simulink model "ltao_v1"  (R2022b)
settings: Solver=FixedStepDiscrete  StartTime=0.0  StopTime=0.6  FixedStep=FEM_Ts  MaxStep=FEM_Ts  RelTol=1e-2
InitFcn:
  | %
  | % Initialization callback function
  | %
  | 
  | try
  |    fprintf('\nGMT IMS version (%s)!\n',simulink_fname );
  | 
  |    % Get Simulink model directory
  |    [filepath,name,ext] = fileparts(which(bdroot));
  | 
  |    if ~strcmp(filepath,pwd)
  |       fprintf('\nChanging current directory to \n %s \n',filepath);
  |       cd(filepath);
  |    end
  | 
  |    %
  |  if(osim.bpless_wl)
  |     fprintf('Generating bumpless wind load time series\n');
  |  end
  | catch
  |    warning('Running the InitFcn from puSimulate script');
  | end
values from neighbouring files (symbols this model uses):
  asm_ssG = XiKL' * asm_ssG * XiKL    [load_ltao_e2e.m]
  Cpi_d = eye(n_Zmodes)* c2d(st.asm.fpi, Ts, c2d_opts)    [evalM2asm_modal.m]    (also in load_ltao_e2e.m = c2d(st.asm.fpi, FEM_Ts, c2d_opts))
  fao_d = c2d(st.glao.fao, st.glao.T, c2d_opts)    [evalM2asm_modal.m]    (also in load_ltao_e2e.m = c2d(st.ltao.fao, FEM_Ts, c2d_opts))
  fao_d4k = c2d(st.ltao.fao, 1/4e3, c2d_opts)    [evalM2asm_modal.m]    (also in load_ltao_e2e.m = c2d(st.ltao.fao, FEM_Ts, c2d_opts))
  FEM_Ts = 1/8e3    (= 0.000125)    [load_ltao_e2e.m]
  fes = c2d(tf((fc_es^2)*4*(pi^2),[1, 2*0.8*fc_es*2*pi, (fc_es^2)*4*(pi^2)]),     st.ltao.T,c2d_opts)    [load_ltao_e2e.m]
  flag_1stOdyn_d = tf(c2d(flag(2,1), Ts, c2d_opts))    [evalM2asm_modal.m]    (also in load_ltao_e2e.m = tf(c2d(flag(2,1),FEM_Ts,c2d_opts)))
  flag_2ndOdyn_d = tf(c2d(flag(3,1), Ts, c2d_opts))    [evalM2asm_modal.m]    (also in load_ltao_e2e.m = tf(c2d(flag(3,1),FEM_Ts,c2d_opts)))
  fpre_d = tf(c2d(st.asm.fpre, Ts, c2d_opts))    [evalM2asm_modal.m]    (also in load_ltao_e2e.m = tf(c2d(fpre,FEM_Ts,c2d_opts)))
  gtt2mnt = eye(2)/(rbm2gtt * Hk_mnt_m1m2)    [load_ltao_e2e.m]
  Hk_mnt_m1m2 = Cm1m2*pinv(Cmnt)    [load_ltao_e2e.m]
  Hpd_d = eye(n_Zmodes)* c2d(st.asm.fpd, Ts, c2d_opts)    [evalM2asm_modal.m]    (also in load_ltao_e2e.m = c2d(st.asm.fpd, FEM_Ts, 'Tustin'))
  Km1rbm_es = (KhpF2es/KhpF2m1rbm)    [load_ltao_e2e.m]
  Ks = cell(7,1)    [load_ltao_e2e.m]
  m1m2_segP_dist = [zeros(42,1); 1e-5*randn(42,1)]    [load_ltao_e2e.m]
  PG = zeros(length(om2),6)    [evalM2asm_modal.m]    (also in load_ltao_e2e.m)
  phiB = inputs2ModalF(mode_ind_vec,indDesInputs) * KinputT    [load_ltao_e2e.m]
  phiC = KoutputT * modalDisp2Outputs(indDesOutputs,mode_ind_vec)    [load_ltao_e2e.m]
  Psi_ss = KoutputT *gainMatrix(indDesOutputs,indDesInputs)* KinputT - K_ss    [load_ltao_e2e.m]
  segPTT2asmCMD = cell(7,1)    [load_ltao_e2e.m]
  Sm1m2_gtt = (Hk_mnt_m1m2*gtt2mnt) * rbm2gtt    [load_ltao_e2e.m]
  st = getcontrol_asm()    [evalM2asm_modal.m]    (also in load_ltao_e2e.m)
undefined symbols (not defined in the file or in its folder): a, az, az_ff_en, b, c, D_seg_piston, D_seg_tt, DiscIntNeverNeededParam, el, fem, gir, m1sys, m2_rbm_dist, m2pos, magnitude, mount, osim, rbm2gtt, Rm1es, Rm2es, sm, VC_modal_stiff
libraries: ims_block_library x7, simulink x2
(part 3 of 3)

== system ltao_v1/Mount_Drv_PDR2021_linear/GIR DT Lugre Fr model/v2z ==
  v : Inport
  g(v) : Inport  Port=2
  z : Inport  Port=3
  Abs : Abs  SaturateOnIntegerOverflow=off
  Divide : Product  Inputs=*/*
  Sum : Sum  Inputs=|+-
  dz : Outport  VectorParamsAs1DForOutWhenUnconnected=off
  wires:
  Abs/1 -> Divide/1
  Divide/1 -> Sum/2
  v/1 -> Sum/1, Abs/1
  Sum/1 -> dz/1
  g(v)/1 -> Divide/2
  z/1 -> Divide/3

== system ltao_v1/Mount_Drv_PDR2021_linear/Parasitic torques model /AZ_Parasitic_Torque ==
  Drive_Pos : Inport
  Drive_Torque : Inport  Port=2
  Cogging : Lookup_n-D  NumberOfTableDimensions=1  LookupTableObject=F_ripple  BreakpointsForDimension1=ParasiticModelStruc.Pos  Table=ParasiticModelStruc.oCog.Amp  InternalRulePriority=Speed  RndMeth=Simplest
  Constant : Constant  Value=0.1869
  Divide : Product  Inputs=**
  EMF Distortion : Lookup_n-D  NumberOfTableDimensions=1  LookupTableObject=F_ripple  BreakpointsForDimension1=ParasiticModelStruc.Pos  Table=ParasiticModelStruc.oEmf.Amp  InternalRulePriority=Speed  RndMeth=Simplest
  Gain : Gain  Gain=1/ParasiticModelStruc.R
  Gain1 : Gain  Gain=1/250
  Gain2 : Gain  Gain=1/ParasiticModelStruc.N_Segm
  Mod : Math  Operator=rem  SignedPower=on
  Mod1 : Math  Operator=rem  SignedPower=on
  Radius : Gain  Gain=ParasiticModelStruc.R
  Sum1 : Sum
  Sum2 : Sum
  Parasitic_Torque : Outport  VectorParamsAs1DForOutWhenUnconnected=off
  wires:
  Divide/1 -> Sum1/1
  Gain1/1 -> Gain2/1  "I_rms"
  Mod1/1 -> EMF Distortion/1, Cogging/1
  Cogging/1 -> Sum1/2
  Radius/1 -> Mod/1  "driven  distance"
  Drive_Torque/1 -> Gain/1
  Gain/1 -> Gain1/1  "Force"
  EMF Distortion/1 -> Divide/2
  Sum2/1 -> Mod1/1
  Mod/1 -> Sum2/1
  Gain2/1 -> Divide/1  "I_rms pro Segment"
  Constant/1 -> Mod/2, Sum2/2, Mod1/2
  Drive_Pos/1 -> Radius/1  "Drive Position"
  Sum1/1 -> Parasitic_Torque/1

== system ltao_v1/Mount_Drv_PDR2021_linear/Parasitic torques model /EL_Parasitic_Torque ==
  Drive_Pos : Inport
  Drive_Torque : Inport  Port=2
  Cogging : Lookup_n-D  NumberOfTableDimensions=1  LookupTableObject=F_ripple  BreakpointsForDimension1=ParasiticModelStruc.Pos  Table=ParasiticModelStruc.oCog.Amp  InternalRulePriority=Speed  RndMeth=Simplest
  Constant : Constant  Value=0.1869
  Divide : Product  Inputs=**
  EMF Distortion : Lookup_n-D  NumberOfTableDimensions=1  LookupTableObject=F_ripple  BreakpointsForDimension1=ParasiticModelStruc.Pos  Table=ParasiticModelStruc.oEmf.Amp  InternalRulePriority=Speed  RndMeth=Simplest
  Gain : Gain  Gain=1/ParasiticModelStruc.R
  Gain1 : Gain  Gain=1/250
  Gain2 : Gain  Gain=1/ParasiticModelStruc.N_Segm
  Mod : Math  Operator=rem  SignedPower=on
  Mod1 : Math  Operator=rem  SignedPower=on
  Radius : Gain  Gain=ParasiticModelStruc.R
  Sum1 : Sum
  Sum2 : Sum
  Parasitic_Torque : Outport  VectorParamsAs1DForOutWhenUnconnected=off
  wires:
  Sum1/1 -> Parasitic_Torque/1
  Drive_Torque/1 -> Gain/1
  EMF Distortion/1 -> Divide/2
  Drive_Pos/1 -> Radius/1  "Drive Position"
  Gain1/1 -> Gain2/1  "I_rms"
  Gain2/1 -> Divide/1  "I_rms pro Segment"
  Gain/1 -> Gain1/1  "Force"
  Mod/1 -> Sum2/1
  Cogging/1 -> Sum1/2
  Radius/1 -> Mod/1  "driven  distance"
  Sum2/1 -> Mod1/1
  Mod1/1 -> EMF Distortion/1, Cogging/1
  Divide/1 -> Sum1/1
  Constant/1 -> Mod/2, Sum2/2, Mod1/2

== system ltao_v1/Mount_Drv_PDR2021_linear/Parasitic torques model /GIR_Parasitic_Torque ==
  note: EMF Torque Model
  note: Cogging Torque Model
  Drive_Pos : Inport
  Drive_Torque : Inport  Port=2
  CogAmp : Constant  Value=ParasiticModelStruc.oCog.amp
  CogSpatFreq : Constant  Value=ParasiticModelStruc.oCog.sfr
  Product : Product
  Product1 : Product  RndMeth=Zero
  Product2 : Product  Inputs=3  RndMeth=Zero
  Product3 : Product  RndMeth=Zero
  Product4 : Product  RndMeth=Zero
  RippleAmpFactor : Constant  Value=ParasiticModelStruc.oEmf.ampFact
  RippleSpatFreq : Constant  Value=ParasiticModelStruc.oEmf.sfr
  Sign : Signum
  Sum : Sum  Inputs=|++
  Sum1 : Sum  Inputs=++|
  ToPretension : Constant  Value=T_pretension
  Trigonometric Function : Trigonometry
  Trigonometric Function1 : Trigonometry
  Parasitic_Torque : Outport  VectorParamsAs1DForOutWhenUnconnected=off
  wires:
  RippleAmpFactor/1 -> Product2/2
  Product1/1 -> Trigonometric Function/1
  RippleSpatFreq/1 -> Product1/2
  Product3/1 -> Trigonometric Function1/1
  Trigonometric Function1/1 -> Product4/1
  CogSpatFreq/1 -> Product3/2
  Drive_Pos/1 -> Product3/1, Product1/1  "Drive Position"
  CogAmp/1 -> Product4/2
  Product4/1 -> Sum/2
  Product2/1 -> Sum/1
  Sum/1 -> Parasitic_Torque/1
  Trigonometric Function/1 -> Product2/3
  Sum1/1 -> Product2/1
  Drive_Torque/1 -> Sign/1, Sum1/2  "Drive Torque (Nm)"
  Sign/1 -> Product/2
  ToPretension/1 -> Product/1
  Product/1 -> Sum1/1

== system ltao_v1/Mount_Drv_PDR2021_linear/Parasitic torques model /Subsystem ==
  Az Pos : Inport
  Az To : Inport  Port=2
  El Pos : Inport  Port=3
  El To : Inport  Port=4
  Gir Pos : Inport  Port=5
  Gir To : Inport  Port=6
  Constant2 : Constant
  Demux1 : Demux  Outputs=3
  Mux1 : Mux  Inputs=3
  Mux7 : Mux  Inputs=3
  Parasitic Torques : Subsystem
  Out1 : Outport  VectorParamsAs1DForOutWhenUnconnected=off
  Out2 : Outport  Port=2  VectorParamsAs1DForOutWhenUnconnected=off
  Out3 : Outport  Port=3  VectorParamsAs1DForOutWhenUnconnected=off
  wires:
  Demux1/1 -> Out1/1
  Demux1/2 -> Out2/1
  Gir Pos/1 -> Mux7/3
  Demux1/3 -> Out3/1
  Az Pos/1 -> Mux7/1
  Mux7/1 -> Parasitic Torques/2(MotPos)
  Mux1/1 -> Parasitic Torques/1(MotTo)
  Constant2/1 -> Parasitic Torques/Enable
  El Pos/1 -> Mux7/2
  Parasitic Torques/1(ParasiticTo) -> Demux1/1
  Az To/1 -> Mux1/1
  El To/1 -> Mux1/2
  Gir To/1 -> Mux1/3

== system ltao_v1/Telescope model/Structural Dynamics GMT/FEM_SS ==
  note: 2nd order form simulation
  In : Inport
  Mount vel gnd : Terminator  Commented=on
  Sum2 : Sum  Inputs=+++
  Sum3 : Sum  Inputs=+++
  Unit Delay : UnitDelay  SampleTime=FEM_Ts  HasFrameUpgradeWarning=on
  Unit Delay1 : UnitDelay  SampleTime=FEM_Ts  HasFrameUpgradeWarning=on
  gamma1 : Gain  Gain=PG(:,3)
  gamma2 : Gain  Gain=PG(:,6)
  phi11 : Gain  Gain=PG(:,1)
  phi12 : Gain  Gain=PG(:,2)
  phi21 : Gain  Gain=PG(:,4)
  phi22 : Gain  Gain=PG(:,5)
  phiB : Gain  Gain=phiB  Multiplication=Matrix(K*u) (u vector)
  phiC : Gain  Gain=phiC  Multiplication=Matrix(K*u) (u vector)
  phiCv : Gain  Gain=phiC(1:14,:)  Multiplication=Matrix(K*u) (u vector)
  pos : Outport  VectorParamsAs1DForOutWhenUnconnected=off
  mount_vel : Outport  Port=2  VectorParamsAs1DForOutWhenUnconnected=off
  wires:
  phiCv/1 -> Mount vel gnd/1, mount_vel/1
  In/1 -> phiB/1
  phiC/1 -> pos/1
  phiB/1 -> gamma1/1, gamma2/1
  Unit Delay1/1 -> phi22/1, phi12/1, phiCv/1
  phi11/1 -> Sum3/3
  gamma1/1 -> Sum3/1
  phi22/1 -> Sum2/1
  phi21/1 -> Sum2/2
  gamma2/1 -> Sum2/3
  Sum3/1 -> Unit Delay/1
  Sum2/1 -> Unit Delay1/1
  phi12/1 -> Sum3/2
  Unit Delay/1 -> phiC/1, phi21/1, phi11/1

== system ltao_v1/Telescope model/Structural Dynamics GMT_/FEM_SS ==
  note: 2nd order form simulation
  In : Inport
  Mount vel gnd : Terminator  Commented=on
  Sum2 : Sum  Inputs=+++
  Sum3 : Sum  Inputs=+++
  Unit Delay : UnitDelay  SampleTime=FEM_Ts  HasFrameUpgradeWarning=on
  Unit Delay1 : UnitDelay  SampleTime=FEM_Ts  HasFrameUpgradeWarning=on
  gamma1 : Gain  Gain=PG(:,3)
  gamma2 : Gain  Gain=PG(:,6)
  phi11 : Gain  Gain=PG(:,1)
  phi12 : Gain  Gain=PG(:,2)
  phi21 : Gain  Gain=PG(:,4)
  phi22 : Gain  Gain=PG(:,5)
  phiB : Gain  Gain=phiB  Multiplication=Matrix(K*u) (u vector)
  phiC : Gain  Gain=phiC  Multiplication=Matrix(K*u) (u vector)
  phiCv : Gain  Gain=phiC(1:14,:)  Multiplication=Matrix(K*u) (u vector)
  pos : Outport  VectorParamsAs1DForOutWhenUnconnected=off
  mount_vel : Outport  Port=2  VectorParamsAs1DForOutWhenUnconnected=off
  wires:
  Unit Delay/1 -> phi11/1, phi21/1, phiC/1
  phi12/1 -> Sum3/2
  Sum2/1 -> Unit Delay1/1
  Sum3/1 -> Unit Delay/1
  gamma2/1 -> Sum2/3
  phi21/1 -> Sum2/2
  phi22/1 -> Sum2/1
  gamma1/1 -> Sum3/1
  phi11/1 -> Sum3/3
  Unit Delay1/1 -> phiCv/1, phi12/1, phi22/1
  phiB/1 -> gamma2/1, gamma1/1
  phiC/1 -> pos/1
  In/1 -> phiB/1
  phiCv/1 -> mount_vel/1, Mount vel gnd/1

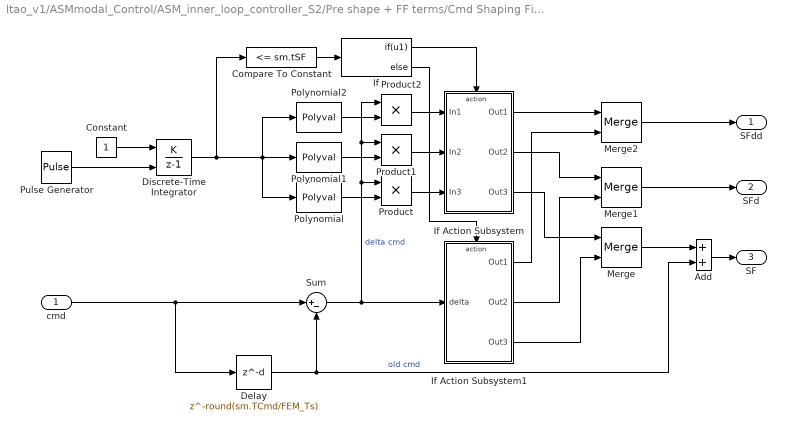
== system ltao_v1/ASMmodal_Control/ASM_inner_loop_controller_S2/Pre shape + FF terms/Cmd Shaping Filter ==
  cmd : Inport
  Add : Sum
  Compare To Constant : simulink/Logic and Bit Operations/Compare To Constant  relop=<=  const=sm.tSF  OutDataTypeStr=boolean
  Constant : Constant
  Delay : Delay  DelayLength=round(sm.TCmd/FEM_Ts)
  Discrete-Time Integrator : DiscreteIntegrator  IntegratorMethod=Accumulation: Forward Euler  gainval=FEM_Ts  ExternalReset=rising  SampleTime=FEM_Ts  ICPrevOutput=DiscIntNeverNeededParam  ICPrevScaledInput=DiscIntNeverNeededParam
  If : If  IfExpression=u1
  If Action Subsystem : Subsystem  TreatAsAtomicUnit=on
  If Action Subsystem1 : Subsystem  TreatAsAtomicUnit=on
  Merge : Merge
  Merge1 : Merge
  Merge2 : Merge
  Polynomial : Polyval  Coefs=[sm.d3SF/20, sm.d2SF/12, sm.d1SF/6, 0, 0, 0]
  Polynomial1 : Polyval  Coefs=[5*sm.d3SF/20, 4*sm.d2SF/12, 3*sm.d1SF/6, 0, 0]
  Polynomial2 : Polyval  Coefs=[20*sm.d3SF/20, 12*sm.d2SF/12, 6*sm.d1SF/6, 0]
  Product : Product
  Product1 : Product
  Product2 : Product
  Pulse Generator : DiscretePulseGenerator  Period=round(sm.TCmd/FEM_Ts)  SampleTime=FEM_Ts
  Sum : Sum  Inputs=|+-
  SFdd : Outport  VectorParamsAs1DForOutWhenUnconnected=off
  SFd : Outport  Port=2  VectorParamsAs1DForOutWhenUnconnected=off
  SF : Outport  Port=3  VectorParamsAs1DForOutWhenUnconnected=off
  wires:
  Discrete-Time Integrator/1 -> Compare To Constant/1, Polynomial2/1, Polynomial/1, Polynomial1/1
  Constant/1 -> Discrete-Time Integrator/1
  Polynomial1/1 -> Product1/2
  Polynomial/1 -> Product/2
  Polynomial2/1 -> Product2/2
  Sum/1 -> If Action Subsystem1/1(delta), Product2/1, Product1/1, Product/1  "delta cmd"
  Add/1 -> SF/1
  Compare To Constant/1 -> If/1
  Product/1 -> If Action Subsystem/3(In3)
  Product1/1 -> If Action Subsystem/2(In2)
  Product2/1 -> If Action Subsystem/1(In1)
  Merge1/1 -> SFd/1
  Merge/1 -> Add/1
  Delay/1 -> Sum/2, Add/2  "old cmd"
  If/1 -> If Action Subsystem/Action
  If/2 -> If Action Subsystem1/Action
  Merge2/1 -> SFdd/1
  If Action Subsystem/1(Out1) -> Merge2/1
  If Action Subsystem1/1(Out1) -> Merge2/2
  If Action Subsystem/2(Out2) -> Merge1/1
  If Action Subsystem/3(Out3) -> Merge/1
  If Action Subsystem1/2(Out2) -> Merge1/2
  If Action Subsystem1/3(Out3) -> Merge/2
  Pulse Generator/1 -> Discrete-Time Integrator/2
  cmd/1 -> Delay/1, Sum/1

== system ltao_v1/Mount_Drv_PDR2021_linear/AZ DT Lugre Fr model/g(v)/gs ==
  v : Inport
  Enable : EnablePort
  Divide : Product  Inputs=**
  Gain : Gain  Gain=1/frParStruct.vs
  Math Function : Math  SignedPower=on
  Math Function1 : Math  Operator=magnitude^2  SignedPower=on
  Sum : Sum  Inputs=|++
  Unary Minus : UnaryMinus
  gc : Constant  Value=frParStruct.Tc/frParStruct.sigm0
  gs : Constant  Value=(frParStruct.Ts-frParStruct.Tc)/frParStruct.sigm0
  gs(v) : Outport  VectorParamsAs1DForOutWhenUnconnected=off
  wires:
  Math Function/1 -> Divide/1
  gs/1 -> Divide/2
  Math Function1/1 -> Unary Minus/1
  Unary Minus/1 -> Math Function/1
  Gain/1 -> Math Function1/1
  v/1 -> Gain/1
  gc/1 -> Sum/2
  Divide/1 -> Sum/1
  Sum/1 -> gs(v)/1

== system ltao_v1/Mount_Drv_PDR2021_linear/EL DT Lugre Fr model/g(v)/gs ==
  v : Inport
  Enable : EnablePort
  Divide : Product  Inputs=**
  Gain : Gain  Gain=1/frParStruct.vs
  Math Function : Math  SignedPower=on
  Math Function1 : Math  Operator=magnitude^2  SignedPower=on
  Unary Minus : UnaryMinus
  gs : Constant  Value=(frParStruct.Ts-frParStruct.Tc)/frParStruct.sigm0
  gs(v) : Outport  VectorParamsAs1DForOutWhenUnconnected=off
  wires:
  Math Function/1 -> Divide/1
  gs/1 -> Divide/2
  Math Function1/1 -> Unary Minus/1
  Unary Minus/1 -> Math Function/1
  Gain/1 -> Math Function1/1
  v/1 -> Gain/1
  Divide/1 -> gs(v)/1

== system ltao_v1/Mount_Drv_PDR2021_linear/GIR DT Lugre Fr model/g(v)/gs ==
  v : Inport
  Enable : EnablePort
  Divide : Product  Inputs=**
  Gain : Gain  Gain=1/frParStruct.vs
  Math Function : Math  SignedPower=on
  Math Function1 : Math  Operator=magnitude^2  SignedPower=on
  Unary Minus : UnaryMinus
  gs : Constant  Value=(frParStruct.Ts-frParStruct.Tc)/frParStruct.sigm0
  gs(v) : Outport  VectorParamsAs1DForOutWhenUnconnected=off
  wires:
  Math Function/1 -> Divide/1
  gs/1 -> Divide/2
  Math Function1/1 -> Unary Minus/1
  Unary Minus/1 -> Math Function/1
  Gain/1 -> Math Function1/1
  v/1 -> Gain/1
  Divide/1 -> gs(v)/1

== system ltao_v1/Mount_Drv_PDR2021_linear/Parasitic torques model /Subsystem/Parasitic Torques ==
  MotTo : Inport
  MotPos : Inport  Port=2
  Enable : EnablePort
  Demux1 : Demux  Outputs=2
  Demux2 : Demux  Outputs=2
  Demux3 : Demux  Outputs=2
  Mux2 : Mux  Inputs=2
  Mux3 : Mux  Inputs=3
  Parasitic AZ : Subsystem  mask{Pos=az.oParasitic.Pos, Amp_Cog=az.oParasitic.oCog.Amp, Amp_EMF=az.oParasitic.oEmf.Amp, R=az.oParasitic.R, N_Segm=az.oParasitic.N_Segm}
  Parasitic EL : Subsystem  mask{Pos=el.oParasitic.Pos, Amp_Cog=el.oParasitic.oCog.Amp, Amp_EMF=el.oParasitic.oEmf.Amp, R=el.oParasitic.R, N_Segm=el.oParasitic.N_Segm}
  Parasitic GIR : Subsystem  mask{cog_sfr=gir.oParasitic.oCog.sfr, cog_amp=gir.oParasitic.oCog.amp, emf_sfr=gir.oParasitic.oEmf.sfr, emf_ampFact=gir.oParasitic.oEmf.ampFact, T_pretension=gir.T_pretension}
  Sel : Selector  InputPortWidth=6  IndexOptions=Index vector (dialog)  Indices=[1 4]  OutputSizes=1
  Sel1 : Selector  InputPortWidth=6  IndexOptions=Index vector (dialog)  Indices=[2 5]  OutputSizes=1
  Sel2 : Selector  InputPortWidth=6  IndexOptions=Index vector (dialog)  Indices=[3 6]  OutputSizes=1
  ParasiticTo : Outport
  wires:
  Mux3/1 -> ParasiticTo/1
  Mux2/1 -> Sel/1, Sel2/1, Sel1/1
  MotTo/1 -> Mux2/1
  MotPos/1 -> Mux2/2
  Sel/1 -> Demux3/1
  Demux3/2 -> Parasitic AZ/2(MotPos)
  Parasitic AZ/1(To) -> Mux3/1
  Sel1/1 -> Demux1/1
  Demux1/2 -> Parasitic EL/2(MotPos)
  Parasitic EL/1(To) -> Mux3/2
  Demux2/1 -> Parasitic GIR/1(MotTo)
  Demux2/2 -> Parasitic GIR/2(MotPos)
  Sel2/1 -> Demux2/1
  Demux3/1 -> Parasitic AZ/1(MotTo)
  Demux1/1 -> Parasitic EL/1(MotTo)
  Parasitic GIR/1(To) -> Mux3/3

== system ltao_v1/ASMmodal_Control/ASM_inner_loop_controller_S2/Pre shape + FF terms/Cmd Shaping Filter/If Action Subsystem ==
  In1 : Inport
  In2 : Inport  Port=2
  In3 : Inport  Port=3
  Action Port : ActionPort
  Out1 : Outport  VectorParamsAs1DForOutWhenUnconnected=off
  Out2 : Outport  Port=2  VectorParamsAs1DForOutWhenUnconnected=off
  Out3 : Outport  Port=3  VectorParamsAs1DForOutWhenUnconnected=off
  wires:
  In1/1 -> Out1/1
  In2/1 -> Out2/1
  In3/1 -> Out3/1

== system ltao_v1/ASMmodal_Control/ASM_inner_loop_controller_S2/Pre shape + FF terms/Cmd Shaping Filter/If Action Subsystem1 ==
  delta : Inport
  Action Port : ActionPort
  Gain : Gain  Gain=0
  Out1 : Outport  VectorParamsAs1DForOutWhenUnconnected=off
  Out2 : Outport  Port=2  VectorParamsAs1DForOutWhenUnconnected=off
  Out3 : Outport  Port=3  VectorParamsAs1DForOutWhenUnconnected=off
  wires:
  delta/1 -> Gain/1, Out3/1
  Gain/1 -> Out1/1, Out2/1

== system ltao_v1/Mount_Drv_PDR2021_linear/Parasitic torques model /Subsystem/Parasitic Torques/Parasitic AZ ==
  MotTo : Inport
  MotPos : Inport  Port=2
  Cogging : Lookup_n-D  NumberOfTableDimensions=1  LookupTableObject=F_ripple  BreakpointsForDimension1=Pos  Table=Amp_Cog  InternalRulePriority=Speed  RndMeth=Simplest
  Constant : Constant  Value=0.1869
  Divide : Product  Inputs=**
  EMF Distortion : Lookup_n-D  NumberOfTableDimensions=1  LookupTableObject=F_ripple  BreakpointsForDimension1=Pos  Table=Amp_EMF  InternalRulePriority=Speed  RndMeth=Simplest
  Gain : Gain  Gain=1/R
  Gain1 : Gain  Gain=1/250
  Gain2 : Gain  Gain=1/N_Segm
  Mod : Math  Operator=rem  SignedPower=on
  Mod1 : Math  Operator=rem  SignedPower=on
  Radius : Gain  Gain=R
  Sum : Sum  Inputs=|++
  Sum1 : Sum  Inputs=|++
  To : Outport
  wires:
  Radius/1 -> Mod/1  "driven  distance"
  Constant/1 -> Mod1/2, Sum1/2, Mod/2
  MotPos/1 -> Radius/1
  Sum/1 -> To/1
  Cogging/1 -> Sum/2
  MotTo/1 -> Gain/1
  Gain/1 -> Gain1/1  "Force"
  EMF Distortion/1 -> Divide/2
  Divide/1 -> Sum/1
  Gain2/1 -> Divide/1  "I_rms pro Segment"
  Gain1/1 -> Gain2/1  "I_rms"
  Mod/1 -> Sum1/1
  Sum1/1 -> Mod1/1
  Mod1/1 -> EMF Distortion/1, Cogging/1

== system ltao_v1/Mount_Drv_PDR2021_linear/Parasitic torques model /Subsystem/Parasitic Torques/Parasitic EL ==
  MotTo : Inport
  MotPos : Inport  Port=2
  Cogging : Lookup_n-D  NumberOfTableDimensions=1  LookupTableObject=F_ripple  BreakpointsForDimension1=Pos  Table=Amp_Cog  InternalRulePriority=Speed  RndMeth=Simplest
  Constant : Constant  Value=0.1869
  Divide : Product  Inputs=**
  EMF Distortion : Lookup_n-D  NumberOfTableDimensions=1  LookupTableObject=F_ripple  BreakpointsForDimension1=Pos  Table=Amp_EMF  InternalRulePriority=Speed  RndMeth=Simplest
  Gain : Gain  Gain=1/R
  Gain1 : Gain  Gain=1/250
  Gain2 : Gain  Gain=1/N_Segm
  Mod1 : Math  Operator=rem  SignedPower=on
  Mod2 : Math  Operator=rem  SignedPower=on
  Radius : Gain  Gain=R
  Scope : Scope  Commented=on  NumInputPorts=2
  Sum : Sum  Inputs=|++
  Sum1 : Sum  Inputs=|++
  To : Outport
  wires:
  MotPos/1 -> Radius/1
  Sum/1 -> To/1
  Cogging/1 -> Scope/2, Sum/2
  MotTo/1 -> Gain/1
  Gain/1 -> Gain1/1  "Force"
  EMF Distortion/1 -> Divide/2
  Divide/1 -> Scope/1, Sum/1
  Gain2/1 -> Divide/1  "I_rms pro Segment"
  Gain1/1 -> Gain2/1  "I_rms"
  Sum1/1 -> Mod2/1
  Mod1/1 -> Sum1/1
  Radius/1 -> Mod1/1  "driven distance"
  Constant/1 -> Mod2/2, Sum1/2, Mod1/2
  Mod2/1 -> Cogging/1, EMF Distortion/1

== system ltao_v1/Mount_Drv_PDR2021_linear/Parasitic torques model /Subsystem/Parasitic Torques/Parasitic GIR ==
  MotTo : Inport
  MotPos : Inport  Port=2
  Cogging : Subsystem
  Emf : Subsystem
  Pretention : Constant  Value=T_pretension
  Product2 : Product  RndMeth=Zero
  Scope : Scope  Commented=on  NumInputPorts=2
  Sign : Signum  ZeroCross=off
  Sum1 : Sum  Inputs=|++
  Sum2 : Sum  Inputs=++|
  To : Outport
  wires:
  Sum2/1 -> To/1
  MotPos/1 -> Cogging/1(Po), Emf/2(Po)
  Cogging/1(T_cog) -> Sum2/2
  Emf/1(T_emf) -> Sum2/1
  Sum1/1 -> Emf/1(To)
  Sign/1 -> Product2/1
  Pretention/1 -> Product2/2
  Product2/1 -> Sum1/2
  MotTo/1 -> Sign/1, Sum1/1

== system ltao_v1/Mount_Drv_PDR2021_linear/Parasitic torques model /Subsystem/Parasitic Torques/Parasitic GIR/Cogging ==
  Po : Inport
  CogAmp : Constant  Value=cog_amp
  CogSpatFreq : Constant  Value=cog_sfr
  Product1 : Product  RndMeth=Zero
  Product2 : Product  RndMeth=Zero
  Trigonometric Function : Trigonometry
  T_cog : Outport
  wires:
  Product1/1 -> Trigonometric Function/1
  CogSpatFreq/1 -> Product1/2
  CogAmp/1 -> Product2/2
  Trigonometric Function/1 -> Product2/1
  Po/1 -> Product1/1
  Product2/1 -> T_cog/1

== system ltao_v1/Mount_Drv_PDR2021_linear/Parasitic torques model /Subsystem/Parasitic Torques/Parasitic GIR/Emf ==
  To : Inport
  Po : Inport  Port=2
  EmfAmpFactor : Constant  Value=emf_ampFact
  EmfSpatFreq : Constant  Value=emf_sfr
  Product1 : Product  RndMeth=Zero
  Product2 : Product  Inputs=3  RndMeth=Zero
  Trigonometric Function : Trigonometry
  T_emf : Outport
  wires:
  Product1/1 -> Trigonometric Function/1
  EmfSpatFreq/1 -> Product1/2
  EmfAmpFactor/1 -> Product2/2
  Trigonometric Function/1 -> Product2/1
  Po/1 -> Product1/1
  Product2/1 -> T_emf/1
  To/1 -> Product2/3

== matlab function ltao_v1/ASMmodal_Control/ASM_inner_loop_controller_S2/Pre shape + FF terms/Command Shaping Filter ==
  data: cmdOld input; cmdSFdd output; cmdSFd output; cmd input; t input; Tcmd input; tSF input; d1SF input; d2SF input; d3SF input; cmdSF output
function [cmdSFdd, cmdSFd, cmdSF] = cmdShFilt(cmdOld, cmd, t, Tcmd, tSF, d1SF, d2SF, d3SF) 
    td = Tcmd;
    nDeltat = floor(t/td);
    tStep = t - td*nDeltat;
    fprintf('tStep:%.3g - nDeltat:%g - td:%.3g\n',tStep,nDeltat,td);
    deltaCmd = cmd - cmdOld;
    if tStep > tSF
        cmdSF = deltaCmd + cmdOld;
        cmdSFd = zeros(size(cmd));
        cmdSFdd = zeros(size(cmd));
    else
        cmdSF = (d1SF/6*tStep^3 + d2SF/12*tStep^4 + d3SF/20*tStep^5)*deltaCmd + cmdOld;
        cmdSFd = (3*d1SF/6*tStep^2 + 4*d2SF/12*tStep^3 + 5*d3SF/20*tStep^4)*deltaCmd;
        cmdSFdd = (6*d1SF/6*tStep + 12*d2SF/12*tStep^2 + 20*d3SF/20*tStep^3)*deltaCmd;
    end
